simulink model "vector_control_param"  (R2021b)
settings: Solver=FixedStepDiscrete  StartTime=0.0  StopTime=inf  RelTol=1e-3  EnableMultiTasking=on
values from neighbouring files (symbols this model uses):
  alphac = 2*pi*300    (= 1884.95559215)    [init.m]
  alphas = 0.1*alphac    (= 188.495559215)    [init.m]
  J = 7.061551833333e-6    (= 7.06155183333e-06)    [init.m]
  Ls = 0.2e-3    (= 0.0002)    [init.m]
  max_rate = 100    [init.m]
  min_rate = -100    [init.m]
  p = 8    [Mtpa.m]    (also in init.m = 4)
  PositionOffset = 3.512    [init.m]
  psi_f = single((Ke)/(sqrt(3)*2*pi*1000*p/60))    [init.m]
  PWM_timer_period = (CPU_clock/Sys_clock_div/fsw/2)/4    (= 1250)    [init.m]
  Rs = 0.36    [init.m]
  T_rated = single((3/2)*p*psi_f*I_rated)    [init.m]
  Ts = 1/(4*fsw)    (= 2.5e-05)    [init.m]
  w_Mn = U_m/psi_s/p    [init.m]
undefined symbols (not defined in the file or in its folder): Down, GPTRIP1SEL, GPTRIP2SEL, TZ1, TZ2, Up
libraries: c2802xlib x7, c280xlib x3, c2837xDlib x3, mcbpositiondecoderlib x3, c2000lib x1, simulink x1
settings Model: ExtModeTrigDuration=8  Creator=Urvelo  LastModifiedBy=jussi
settings SolverCC: AlgebraicLoopSolver=TrustRegion  AutoInsertRateTranBlk=on
settings OptimizationCC: DefaultUnderspecifiedDataType=single  EnhancedBackFolding=on  PassReuseOutputArgsAs=Individual arguments  MaxStackSize=1024  OptimizeBlockOrder=speed  DifferentSizesBufferReuse=on  OptimizationCustomize=off  DenormalBehavior=FlushToZero  EfficientTunableParamExpr=on
settings DebuggingCC: ParameterTunabilityLossMsg=error  SFMachineParentedDataDiag=warning
settings HardwareCC: ProdBitPerChar=16  ProdBitPerInt=16  ProdBitPerPointer=32  ProdBitPerSizeT=32  ProdBitPerPtrDiffT=32  ProdLargestAtomicInteger=Integer  ProdLargestAtomicFloat=None  ProdWordSize=16  ProdLongLongMode=on  ProdHWDeviceType=Texas Instruments->C2000
settings SFSimCC: MATLABDynamicMemAlloc=off
settings RTWCC: Description=Embedded Coder  SystemTargetFile=ert.tlc  HardwareBoard=TI Delfino F28379D LaunchPad  TemplateMakefile=ert_default_tmf  Toolchain=Texas Instruments Code Composer Studio (C2000)
settings CodeAppCC: ForceParamTrailComments=on  IgnoreCustomStorageClasses=off  OperatorAnnotations=on  SimulinkDataObjDesc=on  SFDataObjDesc=on  InsertBlockDesc=on
settings ERTTargetCC: CodeReplacementLibrary=TI C28x  ExtModeTransport=4  ExtModeStaticAlloc=on  ExtModeStaticAllocSize=10000  ExtModeMexFile=ext_xcp  ExtModeIntrfLevel=Level2 - Open

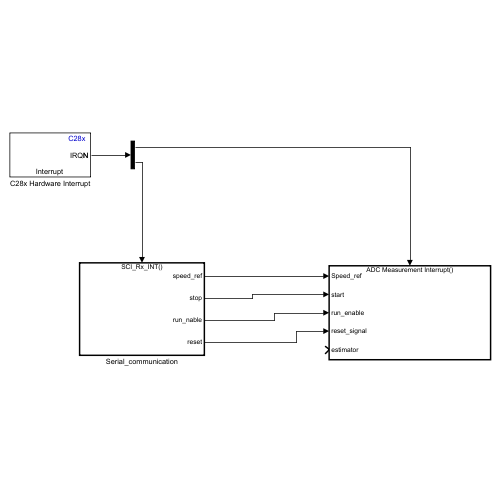
[thumbnail: Simulink's stored preview of the top-level diagram]
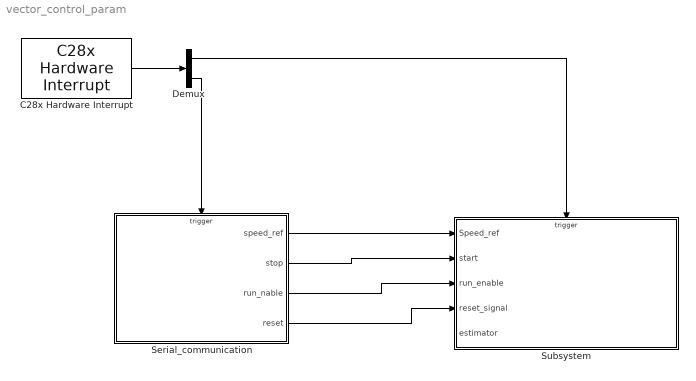
== system vector_control_param ==
  C28x Hardware Interrupt : c2000lib/Scheduling/C28x Hardware Interrupt  irqnumbers=[1 9]  pienumbers=[2 1]  irqpriorities=[30 50]  irqpreempts=[1 0]  showinput=off  dspchiptype=C280X
      settings: SourceProductName=Embedded Coder Support Package for Texas Instruments C2000 Processors
  Demux : Demux  Outputs=2
  Serial_communication : Subsystem
  Subsystem : Subsystem
  wires:
  C28x Hardware Interrupt/1 -> Demux/1
  Demux/2 -> Serial_communication/Trigger
  Demux/1 -> Subsystem/Trigger
  Serial_communication/1(speed_ref) -> Subsystem/1(Speed_ref)
  Serial_communication/2(stop) -> Subsystem/2(start)
  Serial_communication/3(run_nable) -> Subsystem/3(run_enable)
  Serial_communication/4(reset) -> Subsystem/4(reset_signal)

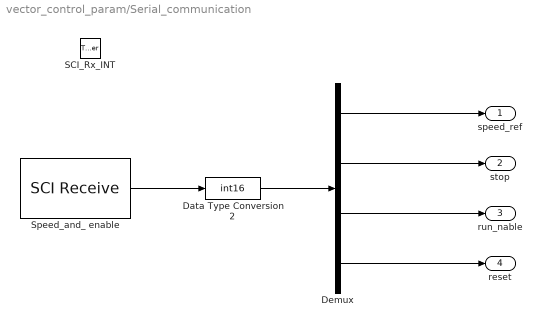
== system vector_control_param/Serial_communication ==
  SCI_Rx_INT : TriggerPort  TriggerType=function-call  VariantControl=Variant
  Data Type Conversion2 : DataTypeConversion  OutDataTypeStr=int16  ConvertRealWorld=Stored Integer (SI)  RndMeth=Simplest
  Demux : Demux
  Speed_and_ enable : c280xlib/SCI Receive  sciModule=A  dataHead=''  dataTail=''  dataType=uint16  dataDim=4  initValue=0  errOption=Output the last received value  errValue=0  sampleTime=-1  outputStatus=off  postInterrupt=on  numFifo=4
      settings: SourceProductName=Embedded Coder Support Package for Texas Instruments C2000 Processors
  speed_ref : Outport
  stop : Outport  Port=2
  run_nable : Outport  Port=3
  reset : Outport  Port=4
  wires:
  Data Type Conversion2/1 -> Demux/1
  Speed_and_ enable/1 -> Data Type Conversion2/1
  Demux/3 -> run_nable/1
  Demux/1 -> speed_ref/1
  Demux/2 -> stop/1
  Demux/4 -> reset/1

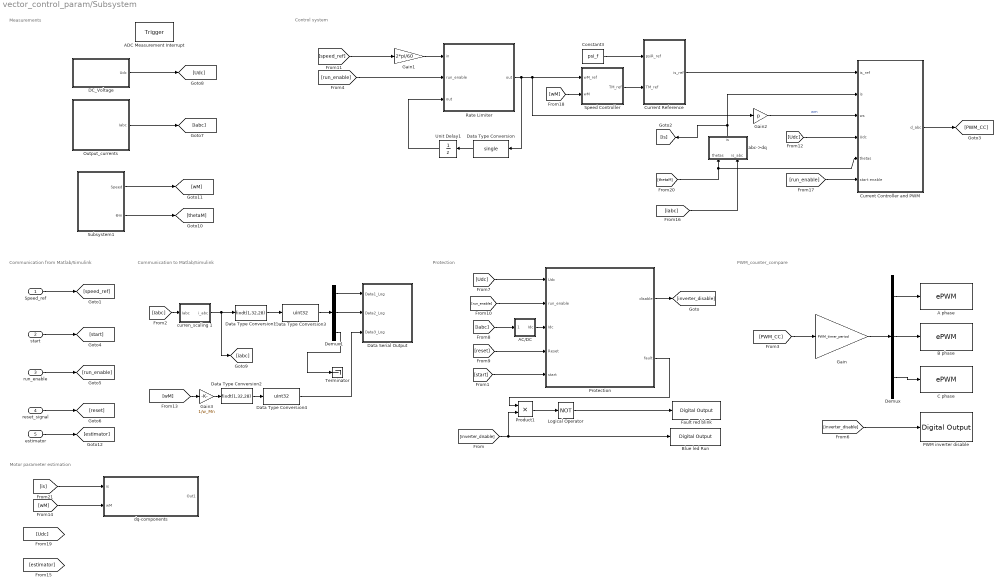
== system vector_control_param/Subsystem ==
  note: Protection
  note: Control system
  note: Communication from Matlab/Simulink
  note: Measurements
  note: Communication to Matlab/Simulink
  note: PWM_counter_compare
  note: Motor parameter estimation
  Speed_ref : Inport
  start : Inport  Port=2
  run_enable : Inport  Port=3
  reset_signal : Inport  Port=4
  estimator : Inport  Port=5
  ADC Measurement Interrupt : TriggerPort  TriggerType=function-call  VariantControl=Variant
  A phase : c2802xlib/ePWM  PwmType=C2000_Type4  useModule=ePWM1  ePWMxLINKTBPRD=Not Linked  periodUnits=Clock cycles  timerSource=Specify via dialog  timerPeriod_clk=PWM_timer_period+1  timerPeriod_sec=0.0001  tbshadow=Counter equals to zero  countingMode=Up-Down  phaseActiveEnable=Disable  phaseDirection=Count down after sync  phaseActive=0  synchronizationEnable=off  dcaevt1Sync=off  dcbevt1Sync=off  synchronizationOption=Counter equals to zero (CTR=Zero)  perSynchronizationOption=Counter equals to period (CTR=PRD)  clockPrescale=1  HSclockPrescale=1  enswap=off  ePWMxAStatus=on  ePWMxAactionLogic1=Do nothing  ePWMxAactionLogic2=Do nothing  ePWMxAactionLogic3=Clear  ePWMxAactionLogic4=Set  ePWMxAactionLogic5=Do nothing  ePWMxAactionLogic6=Do nothing  ePWMxACSFenable=off  ePWMxACSFvalue=Forcing disable  ePWMxASFreload=Zero  ePWMxBStatus=off  ePWMxBactionLogic1=Set  ePWMxBactionLogic2=Clear  ePWMxBactionLogic3=Do nothing  ePWMxBactionLogic4=Do nothing  ePWMxBactionLogic5=Clear  ePWMxBactionLogic6=Set  ePWMxBCSFenable=off  ePWMxBCSFvalue=Forcing disable  ePWMxBSFreload=Zero  ePWNxBOutWay=off  ePWMxLINKCMPA=Not Linked  CMPAUnits=Clock cycles  CMPASource=Input port  CMPAValue_per=50  CMPAValue_clk=PWM_timer_period/2  enCMPAshadow=Counter equals to zero (CTR=Zero)  ePWMxLINKCMPB=Not Linked  CMPBUnits=Clock cycles  CMPBSource=Specify via dialog  CMPBValue_per=50  CMPBValue_clk=PWM_timer_period/2  enCMPBshadow=Counter equals to zero (CTR=Zero)  ePWMxLINKCMPC=Not Linked  CMPCUnits=Clock cycles  CMPCSource=Specify via dialog  CMPCValue_per=50  CMPCValue_clk=32000  enCMPCshadow=Counter equals to zero (CTR=Zero)  ePWMxLINKCMPD=Not Linked  CMPDUnits=Clock cycles  CMPDSource=Specify via dialog  CMPDValue_per=50  CMPDValue_clk=32000  enCMPDshadow=Counter equals to zero (CTR=Zero)  enableDBePWMxA=on  enableDBePWMxB=on  enhalfcycle=off  DBpolarity=Active high complementary (AHC)  DBedgeDelay=Positive  DBSource_ePWMxA=ePWMxA  DBSource_ePWMxB=ePWMxA  DBPeriodUnits=Clock cycles  DBperiodSource=Specify via dialog  REDperiod=15  FEDperiod=15  REDperiod_sec=0  FEDperiod_sec=0  LoadModeDBRED=Immediate without using shadow  LoadModeDBFED=Immediate without using shadow  adcstartModuleA=on  adcrequestEventA=First event  adcstartEventA=Digital Compare Module A Event 1 start of conversion (DCAEVT1.soc)  adcstartEventA_type2=Counter equals to period (CTR=PRD)  adcstartModuleB=off  adcrequestEventB=First event  adcstartEventB=Counter equals to zero (CTR=Zero)  adcstartEventB_type2=Counter equals to zero (CTR=Zero)  intEn=off  intPrd=First event  intSel=Counter equals to zero (CTR=Zero)  intSel_type2=Counter equals to zero (CTR=Zero)  hrpe=off  enHRPWM=off  HRPWM_LoadMode=Counter equals to period (CTR=PRD)  HRPWM_CTLMode=Duty or Period control mode  HRPWM_EDGMode=Both edge  hrpeb=off  enHRPWMB=off  HRPWM_LoadModeB=Counter equals to zero (CTR=ZERO)  HRPWM_CTLModeB=Duty or Period control mode  HRPWM_EDGModeB=Both edge  enHRDBRED=off  enHRDBFED=off  enSFO=on  enautoconv=on  chopperEnable=off  chopperFrequency=1  chopperFirstwidth=1  chopperDuty=12.5%  tripZonesource=Specify via dialog  tzselOSHT1=off  tzselOSHT2=off  tzselOSHT3=off  tzselOSHDCAEV1=off  tzselOSHDCBEV1=off  tzselCBC1=off  tzselCBC2=off  tzselCBC3=off  tzselCBCDCAEV2=off  tzselCBCDCBEV2=off  tzselOSHT4=off  tzselOSHT5=off  tzselOSHT6=off  tzselCBC4=off  tzselCBC5=off  tzselCBC6=off  enTzOstIntr=off  enTzCbcIntr=off  enTzDCAEVT1Intr=off  enTzDCAEVT2Intr=off  enTzDCBEVT1Intr=off  enTzDCBEVT2Intr=off  ePWMxAforced=No action  ePWMxBforced=No action  DCAEVT1forced=No action  DCBEVT1forced=No action  DCAEVT2forced=No action  DCBEVT2forced=No action  dcah=Trip Zone 1 input (TZ1)  dcal=Trip Zone 2 input (TZ2)  dcbh=Trip Zone 1 input (TZ1)  dcbl=Trip Zone 2 input (TZ2)  dcah_type2=GPTRIP1SEL/(TZ1)  dcal_type2=GPTRIP2SEL/(TZ2)  dcbh_type2=GPTRIP1SEL/(TZ1)  dcbl_type2=GPTRIP2SEL/(TZ2)  gendcaevt1=Event disabled  gendcaevt2=Event disabled  gendcbevt1=Event disabled  gendcbevt2=Event disabled  dcaevt1src=DCAEVT1 with sync  dcaevt2src=DCAEVT2 with sync  dcbevt1src=DCBEVT1 with sync  dcbevt2src=DCBEVT2 with sync  pulsesel=Counter equals to zero (CTR=Zero)  blankinv=off  blankoffset=0  blankwidth=0  evsrcsel=Filtered version of DCAEVT1 (DCAEVT1FILT)  encape=off
      settings: SourceProductName=Embedded Coder Support Package for Texas Instruments C2000 Processors
  "AC/DC " : Subsystem
  B phase : c2802xlib/ePWM  PwmType=C2000_Type4  useModule=ePWM2  ePWMxLINKTBPRD=Not Linked  periodUnits=Clock cycles  timerSource=Specify via dialog  timerPeriod_clk=PWM_timer_period  timerPeriod_sec=0.0001  tbshadow=Counter equals to zero  countingMode=Up-Down  phaseActiveEnable=Set counter to phase value specified via dialog  phaseDirection=Count up after sync  phaseActive=0  synchronizationEnable=off  dcaevt1Sync=off  dcbevt1Sync=off  synchronizationOption=Pass through (EPWMxSYNCI or SWFSYNC)  perSynchronizationOption=Counter equals to period (CTR=PRD)  clockPrescale=1  HSclockPrescale=1  enswap=off  ePWMxAStatus=on  ePWMxAactionLogic1=Do nothing  ePWMxAactionLogic2=Do nothing  ePWMxAactionLogic3=Clear  ePWMxAactionLogic4=Set  ePWMxAactionLogic5=Do nothing  ePWMxAactionLogic6=Do nothing  ePWMxACSFenable=off  ePWMxACSFvalue=Forcing disable  ePWMxASFreload=Zero  ePWMxBStatus=off  ePWMxBactionLogic1=Set  ePWMxBactionLogic2=Clear  ePWMxBactionLogic3=Do nothing  ePWMxBactionLogic4=Do nothing  ePWMxBactionLogic5=Clear  ePWMxBactionLogic6=Set  ePWMxBCSFenable=off  ePWMxBCSFvalue=Forcing disable  ePWMxBSFreload=Zero  ePWNxBOutWay=off  ePWMxLINKCMPA=Not Linked  CMPAUnits=Clock cycles  CMPASource=Input port  CMPAValue_per=50  CMPAValue_clk=PWM_timer_period/2  enCMPAshadow=Counter equals to zero (CTR=Zero)  ePWMxLINKCMPB=Not Linked  CMPBUnits=Clock cycles  CMPBSource=Specify via dialog  CMPBValue_per=50  CMPBValue_clk=PWM_timer_period/2  enCMPBshadow=Counter equals to zero (CTR=Zero)  ePWMxLINKCMPC=Not Linked  CMPCUnits=Clock cycles  CMPCSource=Specify via dialog  CMPCValue_per=50  CMPCValue_clk=32000  enCMPCshadow=Counter equals to zero (CTR=Zero)  ePWMxLINKCMPD=Not Linked  CMPDUnits=Clock cycles  CMPDSource=Specify via dialog  CMPDValue_per=50  CMPDValue_clk=32000  enCMPDshadow=Counter equals to zero (CTR=Zero)  enableDBePWMxA=on  enableDBePWMxB=on  enhalfcycle=off  DBpolarity=Active high complementary (AHC)  DBedgeDelay=Positive  DBSource_ePWMxA=ePWMxA  DBSource_ePWMxB=ePWMxA  DBPeriodUnits=Clock cycles  DBperiodSource=Specify via dialog  REDperiod=15  FEDperiod=15  REDperiod_sec=0  FEDperiod_sec=0  LoadModeDBRED=Immediate without using shadow  LoadModeDBFED=Immediate without using shadow  adcstartModuleA=off  adcrequestEventA=First event  adcstartEventA=Digital Compare Module A Event 1 start of conversion (DCAEVT1.soc)  adcstartEventA_type2=Digital Compare Module A Event 1 start of conversion (DCAEVT1.soc)  adcstartModuleB=off  adcrequestEventB=First event  adcstartEventB=Counter equals to zero (CTR=Zero)  adcstartEventB_type2=Counter equals to zero (CTR=Zero)  intEn=off  intPrd=First event  intSel=Counter equals to zero (CTR=Zero)  intSel_type2=Counter equals to zero (CTR=Zero)  hrpe=off  enHRPWM=off  HRPWM_LoadMode=Counter equals to period (CTR=PRD)  HRPWM_CTLMode=Duty or Period control mode  HRPWM_EDGMode=Both edge  hrpeb=off  enHRPWMB=off  HRPWM_LoadModeB=Counter equals to zero (CTR=ZERO)  HRPWM_CTLModeB=Duty or Period control mode  HRPWM_EDGModeB=Both edge  enHRDBRED=off  enHRDBFED=off  enSFO=on  enautoconv=on  chopperEnable=off  chopperFrequency=1  chopperFirstwidth=1  chopperDuty=12.5%  tripZonesource=Specify via dialog  tzselOSHT1=off  tzselOSHT2=off  tzselOSHT3=off  tzselOSHDCAEV1=off  tzselOSHDCBEV1=off  tzselCBC1=off  tzselCBC2=off  tzselCBC3=off  tzselCBCDCAEV2=off  tzselCBCDCBEV2=off  tzselOSHT4=off  tzselOSHT5=off  tzselOSHT6=off  tzselCBC4=off  tzselCBC5=off  tzselCBC6=off  enTzOstIntr=off  enTzCbcIntr=off  enTzDCAEVT1Intr=off  enTzDCAEVT2Intr=off  enTzDCBEVT1Intr=off  enTzDCBEVT2Intr=off  ePWMxAforced=No action  ePWMxBforced=No action  DCAEVT1forced=No action  DCBEVT1forced=No action  DCAEVT2forced=No action  DCBEVT2forced=No action  dcah=Trip Zone 1 input (TZ1)  dcal=Trip Zone 2 input (TZ2)  dcbh=Trip Zone 1 input (TZ1)  dcbl=Trip Zone 2 input (TZ2)  dcah_type2=GPTRIP1SEL/(TZ1)  dcal_type2=GPTRIP2SEL/(TZ2)  dcbh_type2=GPTRIP1SEL/(TZ1)  dcbl_type2=GPTRIP2SEL/(TZ2)  gendcaevt1=Event disabled  gendcaevt2=Event disabled  gendcbevt1=Event disabled  gendcbevt2=Event disabled  dcaevt1src=DCAEVT1 with sync  dcaevt2src=DCAEVT2 with sync  dcbevt1src=DCBEVT1 with sync  dcbevt2src=DCBEVT2 with sync  pulsesel=Counter equals to zero (CTR=Zero)  blankinv=off  blankoffset=0  blankwidth=0  evsrcsel=Filtered version of DCAEVT1 (DCAEVT1FILT)  encape=off
      settings: SourceProductName=Embedded Coder Support Package for Texas Instruments C2000 Processors
  Blue led Run : c2837xDlib/Digital Output  GPIO_Number=GPIO24~GPIO31  GPIO_Bit0=off  GPIO_BIT0_Toggle=off  GPIO_Bit1=off  GPIO_BIT1_Toggle=off  GPIO_Bit2=off  GPIO_BIT2_Toggle=off  GPIO_Bit3=off  GPIO_BIT3_Toggle=off  GPIO_Bit4=off  GPIO_BIT4_Toggle=off  GPIO_Bit5=off  GPIO_BIT5_Toggle=off  GPIO_Bit6=off  GPIO_BIT6_Toggle=off  GPIO_Bit7=on  GPIO_BIT7_Toggle=off
      settings: SourceProductBaseCode=TIC2000
  C phase : c2802xlib/ePWM  PwmType=C2000_Type4  useModule=ePWM3  ePWMxLINKTBPRD=Not Linked  periodUnits=Clock cycles  timerSource=Specify via dialog  timerPeriod_clk=PWM_timer_period  timerPeriod_sec=0.0001  tbshadow=Counter equals to zero  countingMode=Up-Down  phaseActiveEnable=Set counter to phase value specified via dialog  phaseDirection=Count up after sync  phaseActive=0  synchronizationEnable=off  dcaevt1Sync=off  dcbevt1Sync=off  synchronizationOption=Disable  perSynchronizationOption=Counter equals to period (CTR=PRD)  clockPrescale=1  HSclockPrescale=1  enswap=off  ePWMxAStatus=on  ePWMxAactionLogic1=Do nothing  ePWMxAactionLogic2=Do nothing  ePWMxAactionLogic3=Clear  ePWMxAactionLogic4=Set  ePWMxAactionLogic5=Do nothing  ePWMxAactionLogic6=Do nothing  ePWMxACSFenable=off  ePWMxACSFvalue=Forcing disable  ePWMxASFreload=Zero  ePWMxBStatus=off  ePWMxBactionLogic1=Set  ePWMxBactionLogic2=Clear  ePWMxBactionLogic3=Do nothing  ePWMxBactionLogic4=Do nothing  ePWMxBactionLogic5=Clear  ePWMxBactionLogic6=Set  ePWMxBCSFenable=off  ePWMxBCSFvalue=Forcing disable  ePWMxBSFreload=Zero  ePWNxBOutWay=off  ePWMxLINKCMPA=Not Linked  CMPAUnits=Clock cycles  CMPASource=Input port  CMPAValue_per=50  CMPAValue_clk=PWM_timer_period/2  enCMPAshadow=Counter equals to zero (CTR=Zero)  ePWMxLINKCMPB=Not Linked  CMPBUnits=Clock cycles  CMPBSource=Specify via dialog  CMPBValue_per=50  CMPBValue_clk=PWM_timer_period/2  enCMPBshadow=Counter equals to zero (CTR=Zero)  ePWMxLINKCMPC=Not Linked  CMPCUnits=Clock cycles  CMPCSource=Specify via dialog  CMPCValue_per=50  CMPCValue_clk=32000  enCMPCshadow=Counter equals to zero (CTR=Zero)  ePWMxLINKCMPD=Not Linked  CMPDUnits=Clock cycles  CMPDSource=Specify via dialog  CMPDValue_per=50  CMPDValue_clk=32000  enCMPDshadow=Counter equals to zero (CTR=Zero)  enableDBePWMxA=on  enableDBePWMxB=on  enhalfcycle=off  DBpolarity=Active high complementary (AHC)  DBedgeDelay=Positive  DBSource_ePWMxA=ePWMxA  DBSource_ePWMxB=ePWMxA  DBPeriodUnits=Clock cycles  DBperiodSource=Specify via dialog  REDperiod=15  FEDperiod=15  REDperiod_sec=0  FEDperiod_sec=0  LoadModeDBRED=Immediate without using shadow  LoadModeDBFED=Immediate without using shadow  adcstartModuleA=off  adcrequestEventA=First event  adcstartEventA=Digital Compare Module A Event 1 start of conversion (DCAEVT1.soc)  adcstartEventA_type2=Digital Compare Module A Event 1 start of conversion (DCAEVT1.soc)  adcstartModuleB=off  adcrequestEventB=First event  adcstartEventB=Counter equals to zero (CTR=Zero)  adcstartEventB_type2=Counter equals to zero (CTR=Zero)  intEn=off  intPrd=First event  intSel=Counter equals to zero (CTR=Zero)  intSel_type2=Counter equals to zero (CTR=Zero)  hrpe=off  enHRPWM=off  HRPWM_LoadMode=Counter equals to period (CTR=PRD)  HRPWM_CTLMode=Duty or Period control mode  HRPWM_EDGMode=Both edge  hrpeb=off  enHRPWMB=off  HRPWM_LoadModeB=Counter equals to zero (CTR=ZERO)  HRPWM_CTLModeB=Duty or Period control mode  HRPWM_EDGModeB=Both edge  enHRDBRED=off  enHRDBFED=off  enSFO=on  enautoconv=on  chopperEnable=off  chopperFrequency=1  chopperFirstwidth=1  chopperDuty=12.5%  tripZonesource=Specify via dialog  tzselOSHT1=off  tzselOSHT2=off  tzselOSHT3=off  tzselOSHDCAEV1=off  tzselOSHDCBEV1=off  tzselCBC1=off  tzselCBC2=off  tzselCBC3=off  tzselCBCDCAEV2=off  tzselCBCDCBEV2=off  tzselOSHT4=off  tzselOSHT5=off  tzselOSHT6=off  tzselCBC4=off  tzselCBC5=off  tzselCBC6=off  enTzOstIntr=off  enTzCbcIntr=off  enTzDCAEVT1Intr=off  enTzDCAEVT2Intr=off  enTzDCBEVT1Intr=off  enTzDCBEVT2Intr=off  ePWMxAforced=No action  ePWMxBforced=No action  DCAEVT1forced=No action  DCBEVT1forced=No action  DCAEVT2forced=No action  DCBEVT2forced=No action  dcah=Trip Zone 1 input (TZ1)  dcal=Trip Zone 2 input (TZ2)  dcbh=Trip Zone 1 input (TZ1)  dcbl=Trip Zone 2 input (TZ2)  dcah_type2=GPTRIP1SEL/(TZ1)  dcal_type2=GPTRIP2SEL/(TZ2)  dcbh_type2=GPTRIP1SEL/(TZ1)  dcbl_type2=GPTRIP2SEL/(TZ2)  gendcaevt1=Event disabled  gendcaevt2=Event disabled  gendcbevt1=Event disabled  gendcbevt2=Event disabled  dcaevt1src=DCAEVT1 with sync  dcaevt2src=DCAEVT2 with sync  dcbevt1src=DCBEVT1 with sync  dcbevt2src=DCBEVT2 with sync  pulsesel=Counter equals to zero (CTR=Zero)  blankinv=off  blankoffset=0  blankwidth=0  evsrcsel=Filtered version of DCAEVT1 (DCAEVT1FILT)  encape=off
      settings: SourceProductName=Embedded Coder Support Package for Texas Instruments C2000 Processors
  Constant3 : Constant  Value=psi_f  OutDataTypeStr=double  SampleTime=-1
  Current Controller and PWM : Subsystem
  Current Reference : Subsystem
  DC_Voltage : Subsystem
  Data Serial Output : Subsystem
  Data Type Conversion : DataTypeConversion  OutDataTypeStr=single
  Data Type Conversion1 : DataTypeConversion  OutDataTypeStr=fixdt(1,32,28)  RndMeth=Simplest
  Data Type Conversion2 : DataTypeConversion  OutDataTypeStr=fixdt(1,32,28)  RndMeth=Simplest
  Data Type Conversion3 : DataTypeConversion  OutDataTypeStr=uint32  ConvertRealWorld=Stored Integer (SI)  RndMeth=Simplest
  Data Type Conversion4 : DataTypeConversion  OutDataTypeStr=uint32  ConvertRealWorld=Stored Integer (SI)  RndMeth=Simplest
  Demux : Demux  Outputs=3
  Demux1 : Demux  Outputs=3
  Fault red blink : c2837xDlib/Digital Output  GPIO_Number=GPIO32~GPIO39  GPIO_Bit0=off  GPIO_BIT0_Toggle=off  GPIO_Bit1=off  GPIO_BIT1_Toggle=off  GPIO_Bit2=on  GPIO_BIT2_Toggle=off  GPIO_Bit3=off  GPIO_BIT3_Toggle=off  GPIO_Bit4=off  GPIO_BIT4_Toggle=off  GPIO_Bit5=off  GPIO_BIT5_Toggle=off  GPIO_Bit6=off  GPIO_BIT6_Toggle=off  GPIO_Bit7=off  GPIO_BIT7_Toggle=off
      settings: SourceProductBaseCode=TIC2000
  Gain : Gain  Gain=PWM_timer_period  ParamDataTypeStr=single  OutDataTypeStr=single
  Gain1 : Gain  Gain=2*pi/60  OutDataTypeStr=Inherit: Same as input
  Gain2 : Gain  Gain=p
  Gain3 : Gain  Gain=1/w_Mn
  Logical Operator : Logic  Operator=NOT  AllPortsSameDT=off
  Output_currents : Subsystem
  PWM inverter disable : c2837xDlib/Digital Output  GPIO_Number=GPIO120~GPIO127  GPIO_Bit0=off  GPIO_BIT0_Toggle=off  GPIO_Bit1=off  GPIO_BIT1_Toggle=off  GPIO_Bit2=off  GPIO_BIT2_Toggle=off  GPIO_Bit3=off  GPIO_BIT3_Toggle=off  GPIO_Bit4=on  GPIO_BIT4_Toggle=off  GPIO_Bit5=off  GPIO_BIT5_Toggle=off  GPIO_Bit6=off  GPIO_BIT6_Toggle=off  GPIO_Bit7=off  GPIO_BIT7_Toggle=off
      settings: SourceProductBaseCode=TIC2000
  Product1 : Product
  "Protection " : Subsystem
  Rate Limiter : MATLAB Function  TreatAsAtomicUnit=on
  Speed Controller : Subsystem
  Subsystem1 : Subsystem
  Terminator : Terminator
  Unit Delay1 : UnitDelay  SampleTime=-1  HasFrameUpgradeWarning=on
  abc->dq : Subsystem
  curren_scaling 1 : Subsystem
  dq-components : Subsystem
  wires:
  Unit Delay1/1 -> Rate Limiter/3("out ")
  Gain1/1 -> Rate Limiter/1(in)
  [speed_ref] -> Gain1/1
  Current Controller and PWM/1(d_abc) -> [PWM_CC]
  "Protection "/1(disable) -> [inverter_disable]
  Demux/1 -> A phase/1
  Demux/2 -> B phase/1
  Demux/3 -> C phase/1
  Gain/1 -> Demux/1
  Speed_ref/1 -> [speed_ref]
  start/1 -> [start]
  run_enable/1 -> [run_enable]
  reset_signal/1 -> [reset]
  [run_enable] -> Rate Limiter/2(run_enable)
  [PWM_CC] -> Gain/1
  [start] -> "Protection "/5(start)
  [inverter_disable] -> PWM inverter disable/1
  Output_currents/1(Iabc) -> [Iabc]
  DC_Voltage/1(Udc) -> [Udc]
  [iabc] -> "AC/DC "/1(Iabc)
  [reset] -> "Protection "/4(Reset)
  [run_enable] -> "Protection "/2(run_enable)
  "AC/DC "/1(Idc) -> "Protection "/3(Idc)
  [Udc] -> "Protection "/1(Udc)
  [inverter_disable] -> Product1/2, Blue led Run/1
  Logical Operator/1 -> Fault red blink/1
  "Protection "/2(fault) -> Product1/1
  Product1/1 -> Logical Operator/1
  Subsystem1/2(ϴm) -> [thetaM]
  [Iabc] -> curren_scaling 1/1(Iabc)
  Rate Limiter/1(out) -> Data Type Conversion/1, Gain2/1, Speed Controller/1(wM_ref)
  Gain2/1 -> Current Controller and PWM/3(ws)  "wm"
  Data Type Conversion/1 -> Unit Delay1/1
  Data Type Conversion1/1 -> Data Type Conversion3/1
  curren_scaling 1/1(i_abc) -> [iabc], Data Type Conversion1/1
  Data Type Conversion3/1 -> Demux1/1
  Data Type Conversion2/1 -> Data Type Conversion4/1
  [Udc] -> Current Controller and PWM/4(Udc)
  [iabc] -> abc->dq/2(is_abc)
  [run_enable] -> Current Controller and PWM/6(start enable)
  Demux1/1 -> Data Serial Output/1(Data1_Log)
  Constant3/1 -> Current Reference/1(psiR_ref)
  Speed Controller/1(TM_ref) -> Current Reference/2(TM_ref)
  Current Reference/1(is_ref) -> Current Controller and PWM/1(is_ref)
  [thetaM] -> abc->dq/1(thetas), Current Controller and PWM/5(thetas)
  [wM] -> Speed Controller/2(wM)
  Subsystem1/1(Speed) -> [wM]
  [wM] -> Gain3/1
  Gain3/1 -> Data Type Conversion2/1
  Data Type Conversion4/1 -> Data Serial Output/3(Data3_Log)
  Demux1/2 -> Data Serial Output/2(Data2_Log)
  abc->dq/1(is) -> Current Controller and PWM/2(is), [is]
  Demux1/3 -> Terminator/1
  estimator/1 -> [estimator]
  [is] -> dq-components/1(is)
  [wM] -> dq-components/2(wM)

== system vector_control_param/Subsystem/AC//DC  ==
  Iabc : Inport
  DC current : MATLAB Function  TreatAsAtomicUnit=on
  Idc : Outport
  wires:
  DC current/1(Idc) -> Idc/1  "Idc (0...16.5 A)"
  Iabc/1 -> DC current/1(iabc)

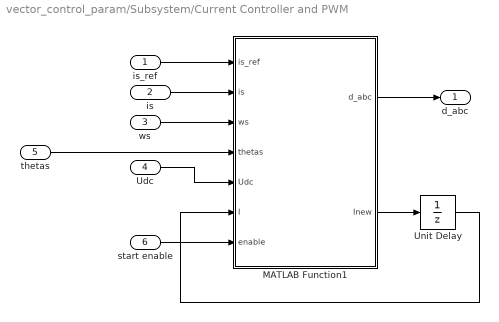
== system vector_control_param/Subsystem/Current Controller and PWM ==
  is_ref : Inport
  is : Inport  Port=2
  ws : Inport  Port=3
  Udc : Inport  Port=4
  thetas : Inport  Port=5
  start enable : Inport  Port=6
  MATLAB Function1 : MATLAB Function  TreatAsAtomicUnit=on
  Unit Delay : UnitDelay  SampleTime=-1  HasFrameUpgradeWarning=on
  d_abc : Outport  PortDimensions=3
  wires:
  MATLAB Function1/2(Inew) -> Unit Delay/1
  ws/1 -> MATLAB Function1/3(ws)
  is/1 -> MATLAB Function1/2(is)
  Udc/1 -> MATLAB Function1/5(Udc)
  MATLAB Function1/1(d_abc) -> d_abc/1
  thetas/1 -> MATLAB Function1/4(thetas)
  Unit Delay/1 -> MATLAB Function1/6(I)
  is_ref/1 -> MATLAB Function1/1(is_ref)
  start enable/1 -> MATLAB Function1/7(enable)

== system vector_control_param/Subsystem/Current Reference ==
  psiR_ref : Inport
  TM_ref : Inport  Port=2
  MATLAB Function : MATLAB Function  TreatAsAtomicUnit=on
  is_ref : Outport
  wires:
  TM_ref/1 -> MATLAB Function/1(TM_ref)
  psiR_ref/1 -> MATLAB Function/2(psi_f)
  MATLAB Function/1(is_ref) -> is_ref/1

== system vector_control_param/Subsystem/DC_Voltage ==
  ADC_C_IN2 : c2802xlib/ADC  blkParamProc=C2000_Type4  ADCModule=A  samplingMode=Single sample mode  ADCResolution=12-bit (Single-ended input)  useSOC1=SOC1  useSOC2=SOC0_SOC1  SOCAcquisitionWindow=15  SOCTriggerSource=ePWM1_ADCSOCA  SOCInterruptTrigger=No ADCINT  Ts=-1  dType=uint16  postInterrupt=off  interruptSel=ADCINT1  ADCINTContinuous=on  endma=off  chdma=1  conv1=ADCINA0  conv2=ADCINA0 and ADCINB0  conv1_Type4=ADCIN14  conv2_Type4=ADCIN0 and ADCIN1
      settings: SourceProductName=Embedded Coder Support Package for Texas Instruments C2000 Processors
  MATLAB Function : MATLAB Function  TreatAsAtomicUnit=on
  Udc : Outport
  wires:
  ADC_C_IN2/1 -> MATLAB Function/1(adc)
  MATLAB Function/1(real) -> Udc/1

== system vector_control_param/Subsystem/Data Serial Output ==
  Data1_Log : Inport
  Data2_Log : Inport  Port=2
  Data3_Log : Inport  Port=3
  Data_Logging : Subsystem
  Demux2 : Demux  Outputs=2
  Mux3 : Mux  Inputs=3
  While Iterator Subsystem : Subsystem  TreatAsAtomicUnit=on
  wires:
  Data2_Log/1 -> Mux3/2  "Offset"
  Data1_Log/1 -> Mux3/1  "Speed"
  Data3_Log/1 -> Mux3/3
  Data_Logging/1(SCI_Tx) -> Demux2/1
  Demux2/1 -> While Iterator Subsystem/1(Data)  "SCI_Tx_Data"
  Demux2/2 -> While Iterator Subsystem/2(Iteration)  "SCI_Tx_Iteration"
  Mux3/1 -> Data_Logging/1(Data_Log)

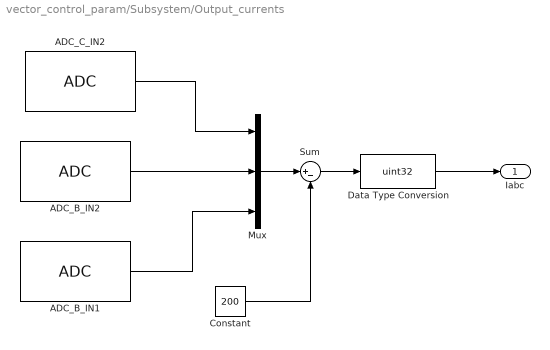
== system vector_control_param/Subsystem/Output_currents ==
  ADC_B_IN1 : c2802xlib/ADC  blkParamProc=C2000_Type4  ADCModule=A  samplingMode=Single sample mode  ADCResolution=12-bit (Single-ended input)  useSOC1=SOC0  useSOC2=SOC0_SOC1  SOCAcquisitionWindow=15  SOCTriggerSource=ePWM1_ADCSOCA  SOCInterruptTrigger=No ADCINT  Ts=-1  dType=uint16  postInterrupt=on  interruptSel=ADCINT1  ADCINTContinuous=on  endma=off  chdma=1  conv1=ADCINA0  conv2=ADCINA0 and ADCINB0  conv1_Type4=ADCIN2  conv2_Type4=ADCIN0 and ADCIN1
      settings: SourceProductName=Embedded Coder Support Package for Texas Instruments C2000 Processors
  ADC_B_IN2 : c2802xlib/ADC  blkParamProc=C2000_Type4  ADCModule=B  samplingMode=Single sample mode  ADCResolution=12-bit (Single-ended input)  useSOC1=SOC0  useSOC2=SOC0_SOC1  SOCAcquisitionWindow=15  SOCTriggerSource=ePWM1_ADCSOCA  SOCInterruptTrigger=No ADCINT  Ts=-1  dType=uint16  postInterrupt=on  interruptSel=ADCINT1  ADCINTContinuous=on  endma=off  chdma=1  conv1=ADCINA0  conv2=ADCINA0 and ADCINB0  conv1_Type4=ADCIN2  conv2_Type4=ADCIN0 and ADCIN1
      settings: SourceProductName=Embedded Coder Support Package for Texas Instruments C2000 Processors
  ADC_C_IN2 : c2802xlib/ADC  blkParamProc=C2000_Type4  ADCModule=C  samplingMode=Single sample mode  ADCResolution=12-bit (Single-ended input)  useSOC1=SOC0  useSOC2=SOC0_SOC1  SOCAcquisitionWindow=15  SOCTriggerSource=ePWM1_ADCSOCA  SOCInterruptTrigger=No ADCINT  Ts=-1  dType=uint16  postInterrupt=off  interruptSel=ADCINT1  ADCINTContinuous=on  endma=off  chdma=1  conv1=ADCINA0  conv2=ADCINA0 and ADCINB0  conv1_Type4=ADCIN2  conv2_Type4=ADCIN0 and ADCIN1
      settings: SourceProductName=Embedded Coder Support Package for Texas Instruments C2000 Processors
  Constant : Constant  Value=200  OutDataTypeStr=uint16  SampleTime=-1
  Data Type Conversion : DataTypeConversion  OutDataTypeStr=uint32  ConvertRealWorld=Stored Integer (SI)
  Mux : Mux  Inputs=3
  Sum : Sum  Inputs=|+-
  Iabc : Outport  InitialOutput=0  VectorParamsAs1DForOutWhenUnconnected=off
  wires:
  ADC_C_IN2/1 -> Mux/1
  ADC_B_IN2/1 -> Mux/2
  ADC_B_IN1/1 -> Mux/3
  Data Type Conversion/1 -> Iabc/1
  Sum/1 -> Data Type Conversion/1
  Mux/1 -> Sum/1
  Constant/1 -> Sum/2

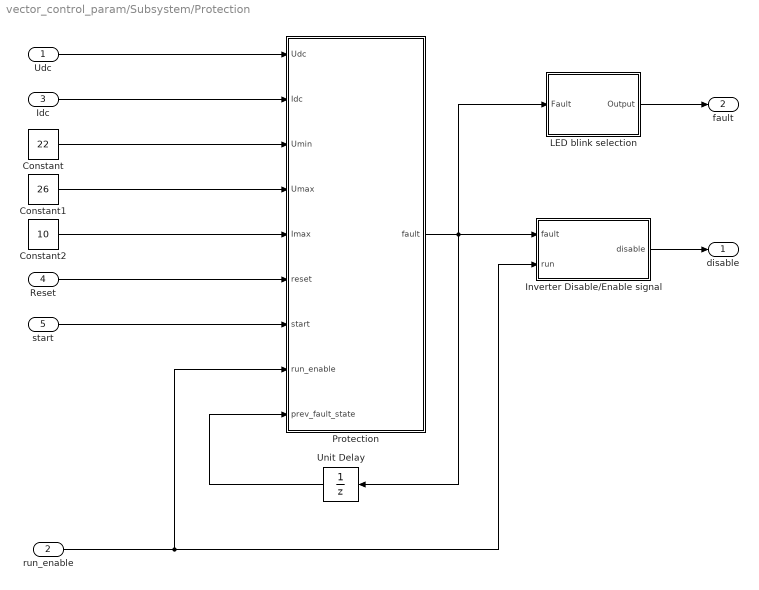
== system vector_control_param/Subsystem/Protection  ==
  Udc : Inport
  run_enable : Inport  Port=2
  Idc : Inport  Port=3
  Reset : Inport  Port=4
  start : Inport  Port=5
  Constant : Constant  Value=22  OutDataTypeStr=single  SampleTime=-1
  Constant1 : Constant  Value=26  OutDataTypeStr=single  SampleTime=-1
  Constant2 : Constant  Value=10  OutDataTypeStr=single  SampleTime=-1
  Inverter Disable/Enable signal : MATLAB Function  TreatAsAtomicUnit=on
  LED blink selection : Subsystem
  Protection : MATLAB Function  TreatAsAtomicUnit=on
  Unit Delay : UnitDelay  SampleTime=-1  HasFrameUpgradeWarning=on
  disable : Outport
  fault : Outport  Port=2
  wires:
  Constant2/1 -> Protection/5(Imax)
  run_enable/1 -> Protection/8(run_enable), Inverter Disable/Enable signal/2(run)
  Unit Delay/1 -> Protection/9(prev_fault_state)
  Constant/1 -> Protection/3(Umin)
  Reset/1 -> Protection/6(reset)
  Constant1/1 -> Protection/4(Umax)
  Inverter Disable/Enable signal/1(disable) -> disable/1
  Udc/1 -> Protection/1(Udc)
  start/1 -> Protection/7(start)
  Idc/1 -> Protection/2(Idc)
  Protection/1(fault) -> LED blink selection/1(Fault), Inverter Disable/Enable signal/1(fault), Unit Delay/1
  LED blink selection/1(Output) -> fault/1

== system vector_control_param/Subsystem/Speed Controller ==
  wM_ref : Inport
  wM : Inport  Port=2
  MATLAB Function : MATLAB Function  TreatAsAtomicUnit=on
  Unit Delay : UnitDelay  SampleTime=-1  HasFrameUpgradeWarning=on
  TM_ref : Outport
  wires:
  wM_ref/1 -> MATLAB Function/1(wM_ref)
  Unit Delay/1 -> MATLAB Function/3(I)
  wM/1 -> MATLAB Function/2(wM)
  MATLAB Function/1(TM_ref_lim) -> TM_ref/1
  MATLAB Function/2(I_new) -> Unit Delay/1

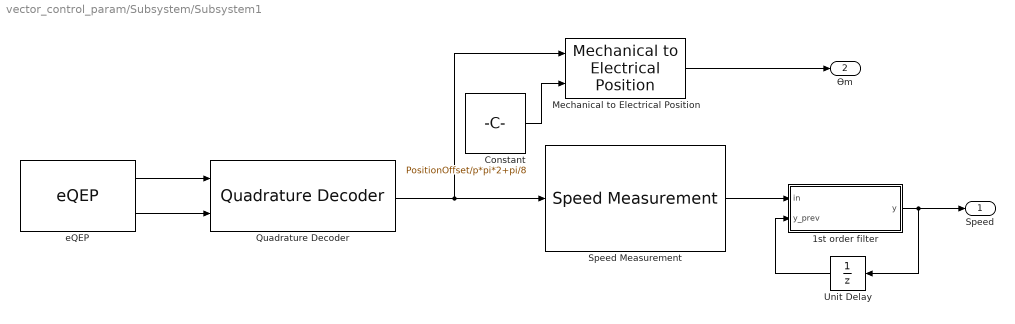
== system vector_control_param/Subsystem/Subsystem1 ==
  1st order filter : MATLAB Function  TreatAsAtomicUnit=on
  Constant : Constant  Value=PositionOffset/p*pi*2+pi/8  SampleTime=-1
  Mechanical to Electrical Position : mcbpositiondecoderlib/Mechanical to Electrical Position  NrPP=p  selectedRange=Radians  MechOfstInputType=Input port  mechOffsetIn=0  maxAngleIn=2*pi  InputDataType=single  VariantSelect=floating-point
      settings: SourceProductBaseCode=MT
  Quadrature Decoder : mcbpositiondecoderlib/Quadrature Decoder  EncoderSlitsPerRevolution=1000  EncoderCountsPerSlit=4  CounterSize=16 bits  ExternalIndexCount=on  PositionUnit=Radians  PositionDataType=single
      settings: SourceProductBaseCode=MT
  Speed Measurement : mcbpositiondecoderlib/Speed Measurement  PositionUnit=Radians  PositionScalingDatatype=uint32  SpeedCalculationMode=Time interval for speed calculation  SampleTimeAsync=Ts  MaximumApplicationSpeed=6000  SpeedResolution=5e-6  DelayLength=20  MaximumMeasurableSpeed=-0.98352  MeasurableSpeedResolution=7.6757e-12  SpeedUnit=Radians/Sec  PerUnitSpeed=6000  SpeedDataType=single
      settings: SourceProductBaseCode=MT
  Unit Delay : UnitDelay  SampleTime=-1  HasFrameUpgradeWarning=on
  eQEP : c280xlib/eQEP  useModule=eQEP1  pcInputmode=Quadrature-count  externalClockrate=2x resolution: Count the rising/falling edge  swapPolarityselection=Clockwise  qdfOutputport=off  qapPolarityselection=on  qbpPolarityselection=on  qipPolarityselection=on  qspPolarityselection=off  igatePolarityselection=off  sampleTime=-1  pcOutputport=on  pcMaximumvalue=2^16- 1  indexInitializationcheck=off  indexInitializationevent=Rising edge  strobeInitializationcheck=off  strobeInitializationevent=Rising edge  softwareInitializationcheck=off  softwareInitializationsource=Set to init value at start up  softwareInitializationmode=on  pcInitialvalue=2147483648  pcResetmode=Reset on the first index event  ieloutputport=on  indexEventlatch=Falling edge  seloutputport=off  strobeEventlatch=Rising edge  pcefOutputport=off  enableEqepcapture=off  qctmrOutputport=off  qcprdOutputport=off  captureTimerprescaler=128  upEventprescaler=128  overflowErrorflag=off  directionErrorflag=off  captureTimerposition=On position counter read  unitTimerperiod=100000000  captureTimerlatch=off  capturePeriodlatch=off  positionCounterlatch=off  soenPolarityselection=off  spselPolarityselection=Index pin is used for sync output  compareValuesource=Specify via dialog  shadowMode=Load on QPOSCNT=0  compareValue=4294967295  syncOutputwidth=1  polaritySyncoutput=Active high  watchdogEnable=off  watchdogTimer=65535  outport1Datatype=auto  outport2Datatype=auto  outport3Datatype=auto  outport4Datatype=auto  outport5Datatype=auto  outport6Datatype=auto  outport7Datatype=auto  outport8Datatype=auto  outport9Datatype=auto  outport10Datatype=auto  outport11Datatype=auto  outport12Datatype=auto  eqepinterrupt_pce=off  eqepinterrupt_qpe=off  eqepinterrupt_qdc=off  eqepinterrupt_wto=off  eqepinterrupt_pcu=off  eqepinterrupt_pco=off  eqepinterrupt_pcr=off  eqepinterrupt_pcm=off  eqepinterrupt_sel=off  eqepinterrupt_iel=off  eqepinterrupt_uto=off  pheOutputport=off  watchdogOutputport=off  outport13Datatype=auto  outport14Datatype=auto
      settings: SourceProductName=Embedded Coder Support Package for Texas Instruments C2000 Processors
  Speed : Outport
  ϴm : Outport  Port=2
  wires:
  eQEP/2 -> Quadrature Decoder/2
  Speed Measurement/1 -> 1st order filter/1(in)
  eQEP/1 -> Quadrature Decoder/1
  Quadrature Decoder/1 -> Mechanical to Electrical Position/1, Speed Measurement/1
  Constant/1 -> Mechanical to Electrical Position/2
  1st order filter/1(y) -> Unit Delay/1, Speed/1
  Mechanical to Electrical Position/1 -> ϴm/1
  Unit Delay/1 -> 1st order filter/2(y_prev)

== system vector_control_param/Subsystem/abc->dq ==
  thetas : Inport
  is_abc : Inport  Port=2
  MATLAB Function : MATLAB Function  TreatAsAtomicUnit=on
  is : Outport
  wires:
  MATLAB Function/1(is) -> is/1
  thetas/1 -> MATLAB Function/2(thetas)
  is_abc/1 -> MATLAB Function/1(is_abc)

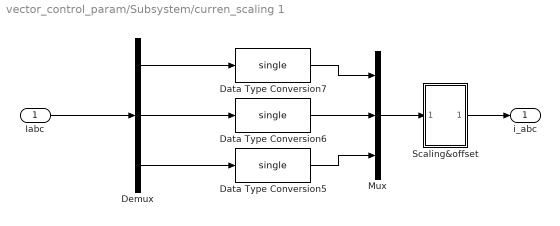
== system vector_control_param/Subsystem/curren_scaling 1 ==
  Iabc : Inport
  Data Type Conversion5 : DataTypeConversion  OutDataTypeStr=single  ConvertRealWorld=Stored Integer (SI)
  Data Type Conversion6 : DataTypeConversion  OutDataTypeStr=single  ConvertRealWorld=Stored Integer (SI)
  Data Type Conversion7 : DataTypeConversion  OutDataTypeStr=single  ConvertRealWorld=Stored Integer (SI)
  Demux : Demux  Outputs=3
  Mux : Mux  Inputs=3
  Scaling&offset : Subsystem
  i_abc : Outport
  wires:
  Iabc/1 -> Demux/1
  Demux/3 -> Data Type Conversion5/1
  Demux/1 -> Data Type Conversion7/1
  Demux/2 -> Data Type Conversion6/1
  Scaling&offset/1(iabc) -> i_abc/1
  Data Type Conversion7/1 -> Mux/1
  Mux/1 -> Scaling&offset/1(In1)
  Data Type Conversion5/1 -> Mux/3
  Data Type Conversion6/1 -> Mux/2

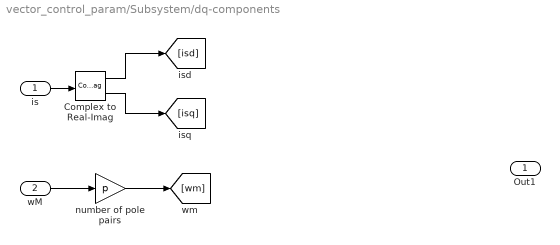
== system vector_control_param/Subsystem/dq-components ==
  is : Inport
  wM : Inport  Port=2
  Complex to Real-Imag : ComplexToRealImag
  number of pole pairs : Gain  Gain=p
  Out1 : Outport
  wires:
  is/1 -> Complex to Real-Imag/1
  Complex to Real-Imag/1 -> [isd]
  Complex to Real-Imag/2 -> [isq]
  wM/1 -> number of pole pairs/1
  number of pole pairs/1 -> [wm]

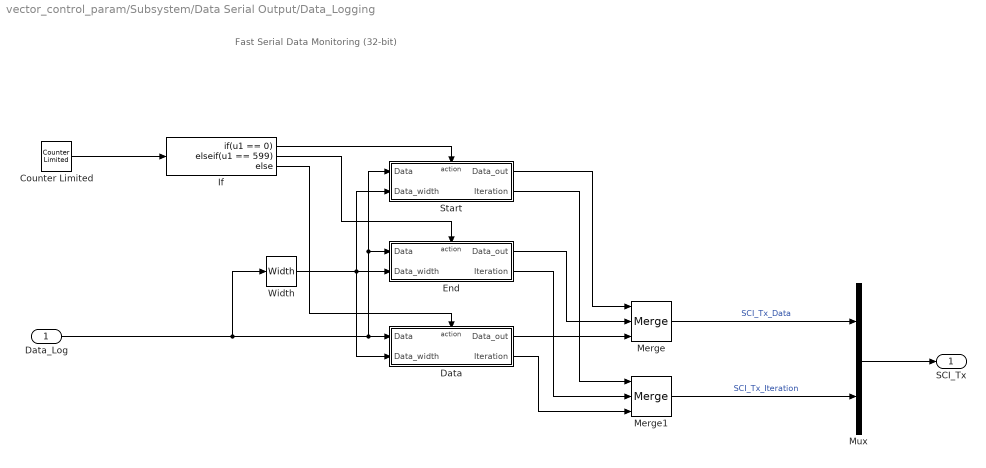
== system vector_control_param/Subsystem/Data Serial Output/Data_Logging ==
  note: Fast Serial Data Monitoring (32-bit)
  Data_Log : Inport
  Counter Limited : simulink/Sources/Counter Limited  uplimit=600-1  tsamp=-1
  Data : Subsystem  TreatAsAtomicUnit=on
  End : Subsystem  TreatAsAtomicUnit=on
  If : If  IfExpression=u1 == 0  ElseIfExpressions=u1 == 599
  Merge : Merge  Inputs=3
  Merge1 : Merge  Inputs=3
  Mux : Mux  Inputs=2
  Start : Subsystem  TreatAsAtomicUnit=on
  Width : Width  OutDataTypeMode=All ports same datatype  DataType=uint16
  SCI_Tx : Outport
  wires:
  If/3 -> Data/Action
  Data/1(Data_out) -> Merge/3
  Width/1 -> Data/2(Data_width), Start/2(Data_width), End/2(Data_width)
  Merge/1 -> Mux/1  "SCI_Tx_Data"
  Counter Limited/1 -> If/1
  Start/2(Iteration) -> Merge1/1
  Start/1(Data_out) -> Merge/1
  If/2 -> End/Action
  Merge1/1 -> Mux/2  "SCI_Tx_Iteration"
  If/1 -> Start/Action
  End/1(Data_out) -> Merge/2
  End/2(Iteration) -> Merge1/2
  Data/2(Iteration) -> Merge1/3
  Mux/1 -> SCI_Tx/1
  Data_Log/1 -> Width/1, Start/1(Data), End/1(Data), Data/1(Data)

== system vector_control_param/Subsystem/Data Serial Output/While Iterator Subsystem ==
  Data : Inport
  Iteration : Inport  Port=2
  Add : Sum  Inputs=+-  OutDataTypeStr=Inherit: Same as first input
  Index Vector : MultiPortSwitch  Inputs=1
  SCI Transmit : c280xlib/SCI Transmit  sciModule=A  dataHead=''  dataTail=''  postInterrupt=off  numFifo=1
      settings: SourceProductName=Embedded Coder Support Package for Texas Instruments C2000 Processors
  While Iterator : WhileIterator  MaxIters=-1  WhileBlockType=do-while  ShowIterationPort=on  OutputDataType=int16
  wires:
  While Iterator/1 -> Add/2, Index Vector/1
  Data/1 -> Index Vector/2
  Index Vector/1 -> SCI Transmit/1
  Add/1 -> While Iterator/1
  Iteration/1 -> Add/1

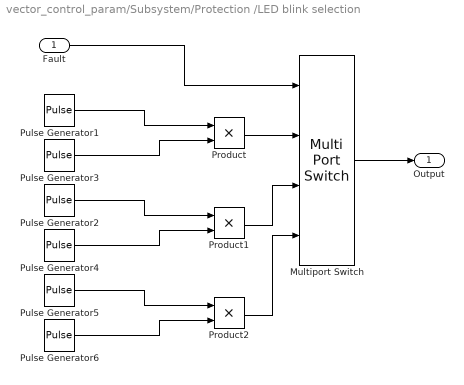
== system vector_control_param/Subsystem/Protection /LED blink selection ==
  Fault : Inport
  Multiport Switch : MultiPortSwitch
  Product : Product
  Product1 : Product
  Product2 : Product
  Pulse Generator1 : DiscretePulseGenerator  Period=15000  PulseWidth=5000  SampleTime=-1
  Pulse Generator2 : DiscretePulseGenerator  Period=20000  PulseWidth=10000  SampleTime=-1
  Pulse Generator3 : DiscretePulseGenerator  Period=5000  PulseWidth=2500  SampleTime=-1
  Pulse Generator4 : DiscretePulseGenerator  Period=5000  PulseWidth=2500  SampleTime=-1
  Pulse Generator5 : DiscretePulseGenerator  Period=25000  PulseWidth=15000  SampleTime=-1
  Pulse Generator6 : DiscretePulseGenerator  Period=5000  PulseWidth=2500  SampleTime=-1
  Output : Outport
  wires:
  Pulse Generator4/1 -> Product1/2
  Product2/1 -> Multiport Switch/4
  Pulse Generator2/1 -> Product1/1
  Pulse Generator3/1 -> Product/2
  Fault/1 -> Multiport Switch/1
  Multiport Switch/1 -> Output/1
  Pulse Generator5/1 -> Product2/1
  Pulse Generator1/1 -> Product/1
  Pulse Generator6/1 -> Product2/2
  Product1/1 -> Multiport Switch/3
  Product/1 -> Multiport Switch/2

== system vector_control_param/Subsystem/curren_scaling 1/Scaling&offset ==
  In1 : Inport
  Constant : Constant  Value=3.3/(5e-3*20*2)  OutDataTypeStr=single
  Gain : Gain  Gain=1/4095*3.3/(5e-3*20)
  Gain1 : Gain  Gain=-1
  Sum : Sum  Inputs=|+-
  iabc : Outport
  wires:
  In1/1 -> Gain/1
  Constant/1 -> Sum/2
  Gain/1 -> Sum/1
  Sum/1 -> Gain1/1
  Gain1/1 -> iabc/1

== system vector_control_param/Subsystem/Data Serial Output/Data_Logging/Data ==
  Data : Inport
  Data_width : Inport  Port=2
  Action Port : ActionPort  ActionPortLabel=else
  Dummy : Constant  Value=hex2dec('0000')  OutDataTypeStr=uint32
  Mux : Mux  Inputs=2
  Data_out : Outport  VectorParamsAs1DForOutWhenUnconnected=off
  Iteration : Outport  Port=2  VectorParamsAs1DForOutWhenUnconnected=off
  wires:
  Data_width/1 -> Iteration/1
  Data/1 -> Mux/1
  Dummy/1 -> Mux/2
  Mux/1 -> Data_out/1

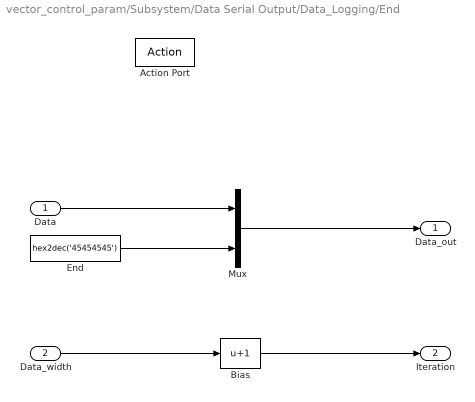
== system vector_control_param/Subsystem/Data Serial Output/Data_Logging/End ==
  Data : Inport
  Data_width : Inport  Port=2
  Action Port : ActionPort  ActionPortLabel=elseif(u1 == 599)
  Bias : Bias  Bias=1
  End : Constant  Value=hex2dec('45454545')  OutDataTypeStr=uint32
  Mux : Mux  Inputs=2
  Data_out : Outport  VectorParamsAs1DForOutWhenUnconnected=off
  Iteration : Outport  Port=2  VectorParamsAs1DForOutWhenUnconnected=off
  wires:
  Data/1 -> Mux/1
  Data_width/1 -> Bias/1
  Bias/1 -> Iteration/1
  End/1 -> Mux/2
  Mux/1 -> Data_out/1

== system vector_control_param/Subsystem/Data Serial Output/Data_Logging/Start ==
  Data : Inport
  Data_width : Inport  Port=2
  Action Port : ActionPort  ActionPortLabel=if(u1 == 0)
  Bias : Bias  Bias=1
  Mux : Mux  Inputs=2
  Start : Constant  Value=hex2dec('53535353')  OutDataTypeStr=uint32
  Data_out : Outport  VectorParamsAs1DForOutWhenUnconnected=off
  Iteration : Outport  Port=2  VectorParamsAs1DForOutWhenUnconnected=off
  wires:
  Data/1 -> Mux/2
  Data_width/1 -> Bias/1
  Bias/1 -> Iteration/1
  Start/1 -> Mux/1
  Mux/1 -> Data_out/1

== matlab function vector_control_param/Subsystem/AC//DC /DC current ==
  data: iabc input; Idc output
function Idc = Clarke(iabc)
ia = iabc(1);
ib = iabc(2);
ic = iabc(3);
is=2/3*(ia+ib*exp(1j*2*pi/3)+ic*exp(1j*4*pi/3));
Idc = abs(is);

== matlab function vector_control_param/Subsystem/Protection /Inverter Disable//Enable signal ==
  data: fault input; disable output; run input
function disable = fcn(fault, run)

% persistent count
% if isempty(count)
% count = 0;
% end

if (fault == 0 && run == 1)
    disable = single(0);
%    count = 0;
else
    disable = single(1);
%     if (fault > 0)
%         if (count < 3)
%             count = count + 1;    
%         end
%     end
%     if (fault == 1 && count == 1)
%         disp('Inverter disabled - Undervoltage protection. Please debug the problem and reset the model.');
%     end
%     if (fault == 2 && count == 1)
%         disp('Inverter disabled - Overvoltage protection. Please debug the problem and reset the model.');
%     end
%     if (fault == 3 && count == 1)
%         disp('Inverter disabled - Overcurrent protection. Please debug the problem and reset the model.');
%     end
end

== matlab function vector_control_param/Subsystem/Current Reference/MATLAB Function ==
  settings: updateMethod=DISCRETE
  data: TM_ref input; psi_f input; p parameter size=1; is_ref output
function is_ref = curr_ref(TM_ref, psi_f, p)

%% Current references in estimated rotor-flux coordinates

iq_ref = 2/(3*p) * TM_ref/psi_f;
id_ref = 0;


is_ref = single(id_ref + 1j*iq_ref);

== matlab function vector_control_param/Subsystem/abc->dq/MATLAB Function ==
  data: is_abc input size=3; thetas input size=1; is output size=1
function is = abc_dq(is_abc, thetas)

% Phase currents
ia = is_abc(1); 
ib = is_abc(2);
ic = is_abc(3); 
% Transformation to alpha beta coordinates
iss = 2/3*(ia + ib*exp(1j*2*pi/3) + ic*exp(1j*4*pi/3));
% Transformation to d-q coordinates
is = single(iss*exp(-1j*thetas));

% alternative formula -> not all MCUs supports imaginary numbers
%ialpha = 2/3*(ia - 1/2*ib - 1/2*ic);
%ibeta = 2/3*(sqrt(3)/2*ib - sqrt(3)/2*ic);
%iss = ialpha +1j*ibeta;
% Space-vector transformation and coordinate transformation
%is = iss*(cos(thetas)-1j*sin(thetas));

== matlab function vector_control_param/Subsystem/Speed Controller/MATLAB Function ==
  data: wM_ref input size=1; wM input size=1; I input size=1; J parameter size=1; alphas parameter size=1; T_rated parameter size=1; TM_ref_lim output; Ts parameter size=1; I_new output
function [TM_ref_lim, I_new] = speed_ctrl(wM_ref, wM, I, J, alphas, T_rated, Ts)

% Speed controller
ba = alphas*J;
kp = alphas*J;
ki = alphas^2*J;

e = wM_ref - wM;
TM_ref = kp*e + ki*I - ba*wM;

% Limited reference
TM_ref_lim = single(TM_ref);
if(TM_ref_lim > T_rated)
    TM_ref_lim = single(T_rated);
elseif(TM_ref_lim < -T_rated)
    TM_ref_lim = single(-T_rated);
end

% Update state
I_new = single(I + Ts*(e + (TM_ref_lim - TM_ref)/kp));

== matlab function vector_control_param/Subsystem/Current Controller and PWM/MATLAB Function1 ==
  data: is_ref input size=1; is input size=1; ws input; thetas input size=1; Udc input size=1; I input size=1; Rs parameter; Ls parameter size=1; alphac parameter size=1; Ts parameter size=1; d_abc output size=3; Inew output; psi_f parameter; enable input
function [d_abc, Inew] = cc(is_ref, is, ws, thetas, Udc, I, Rs, Ls, alphac, Ts, psi_f, enable)
%#codegen


%% Current controller 
% Gains
kp = alphac*Ls;
ki = alphac^2*Ls;
Ra = alphac*Ls - Rs;

% Voltage reference in synchronous coordinates
e = is_ref - is;
us_ref = kp*e + ki*I - Ra*is + 1j*ws*(Ls*is + psi_f);

    
% Reference in stator coordinates
thetasc = thetas + 1.5*Ts*ws;   % Compensation for discrete-time delays
if (enable == 1) 
uss_ref = us_ref*exp(1j*thetasc);
else 
    uss_ref = single(0 + 0*1j);
end

%% Symmetrical suboscillation PWM
% Components of the voltage space vector
ualpha_ref = real(uss_ref);
ubeta_ref  = imag(uss_ref);

% Phase-voltage references
ua_ref = ualpha_ref;
ub_ref = .5*(-ualpha_ref + sqrt(3)*ubeta_ref);
uc_ref = .5*(-ualpha_ref - sqrt(3)*ubeta_ref);

% Vector of phase-voltage references
u_abc_ref = [ua_ref; ub_ref; uc_ref];

% Symmetrization of the references by adding the zero-sequence voltage
u0 = .5*(max(u_abc_ref) + min(u_abc_ref));
u_abc_ref = u_abc_ref - u0;

% Clamping of the reference voltages such that no phase error is caused. 
% If all phase voltage reference are realizable (below Udc/2), m = 1 holds.
Udc = single(Udc) %  Here is the signal variable size changed
m = max([2*u_abc_ref/Udc; 1]);
u_abc_ref = u_abc_ref/m;

% Duty cycles, which can be directly used for triangle comparison, 
% if the triangle wave varies between 0...1
d_abc = single(.5 + u_abc_ref/Udc);

% Realized voltage vector is calculated from the clamped duty ratios.
% If the PWM does not saturate, us_ref_lim = us_ref holds. The realized
% voltage vector is needed, e.g., for the current-controller antiwindup.
uss_ref_lim = single(2/3*(d_abc(1) + d_abc(2)*exp(1j*2*pi/3) + d_abc(3)*exp(1j*4*pi/3))*Udc);
% In estimated rotor flux coordinates
us_ref_lim = single(exp(-1j*thetasc)*uss_ref_lim);  

%% Update the integral state of the current controller 
if (enable == 1) 
Inew = single(I + Ts*(e + (us_ref_lim - us_ref)/kp));
else 
    Inew = single(0+0*1j);
end

== matlab function vector_control_param/Subsystem/Subsystem1/1st order filter ==
  data: in input; y output; y_prev input; a parameter
function y = filter(in, y_prev, a)

y = (1-a)*y_prev + in*a;

== matlab function vector_control_param/Subsystem/Protection /Protection ==
  data: Udc input; fault output; Idc input; Umin input; Umax input; Imax input; reset input; start input; run_enable input; prev_fault_state input
function fault = protection(Udc, Idc, Umin, Umax, Imax, reset, start, run_enable, prev_fault_state)
if (Udc < Umin || Udc > Umax || Idc > Imax)   
    fault = single(1);
else
    fault = prev_fault_state;
end

if (reset == 1 && fault == 1 && start == 0 && run_enable == 0)
   fault = single(0);
end

== matlab function vector_control_param/Subsystem/Rate Limiter ==
  data: in input; run_enable input; out input; out output; max_rate parameter; min_rate parameter; Ts parameter
function out  = fcn(in, run_enable, out, max_rate, min_rate, Ts)
if run_enable == 0
    out = single(0);
end
persistent rate
in = single(in) % Here is the signal variable size changed  
    if isempty(rate)
        rate = (in-out)/Ts;
    else
    rate = (in-out)/Ts;
    end
    if (rate > max_rate)
        out = Ts*max_rate + out;
    elseif (rate < min_rate)
        out = Ts*min_rate + out;
    elseif (rate > min_rate || rate < max_rate)
        out = in;
    end

== matlab function vector_control_param/Subsystem/DC_Voltage/MATLAB Function ==
  data: adc input; real output
function real = fcn(adc)

   x = (adc*80/4095-52/3)/(13/6);
   real =  2.1639*x + 17.337 - 0.1639*x - 1.337;
